simulink model "relay_method_for_id"  (R2017a)
settings: Solver=VariableStepAuto  StartTime=0.0  StopTime=240  RelTol=1e-3
settings Model: Creator=test  LastModifiedBy=test

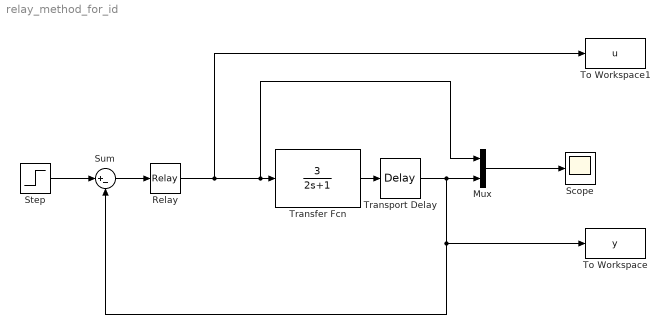
== system relay_method_for_id ==
  Mux : Mux  Inputs=2
  Relay : Relay  OnSwitchValue=0.9  OffSwitchValue=-0.9  OnOutputValue=1.5  OffOutputValue=-0.5
  Scope : Scope
  Step : Step  Time=3  After=2  SampleTime=0
  Sum : Sum  Inputs=|+-
  To Workspace : ToWorkspace  VariableName=y  SaveFormat=Timeseries  SampleTime=-1
  To Workspace1 : ToWorkspace  VariableName=u  SaveFormat=Timeseries  SampleTime=-1
  Transfer Fcn : TransferFcn  Numerator=[3]  Denominator=[2 1]
  Transport Delay : TransportDelay  DelayTime=0.1
  wires:
  Transfer Fcn/1 -> Transport Delay/1
  Relay/1 -> To Workspace1/1, Mux/1, Transfer Fcn/1
  Mux/1 -> Scope/1
  Step/1 -> Sum/1
  Sum/1 -> Relay/1
  Transport Delay/1 -> Mux/2, To Workspace/1, Sum/2
